simulink model "untitled"  (R2023a)
settings: Solver=daessc  StartTime=0.0  StopTime=15  MaxStep=1e-7  RelTol=1e-3
settings Model: Creator=alexey  LastModifiedBy=alexey

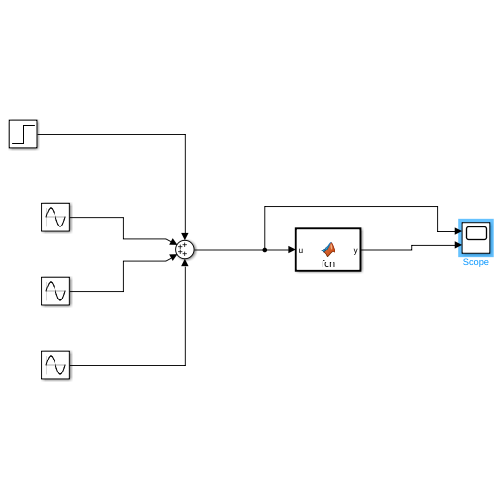
[thumbnail: Simulink's stored preview of the top-level diagram]
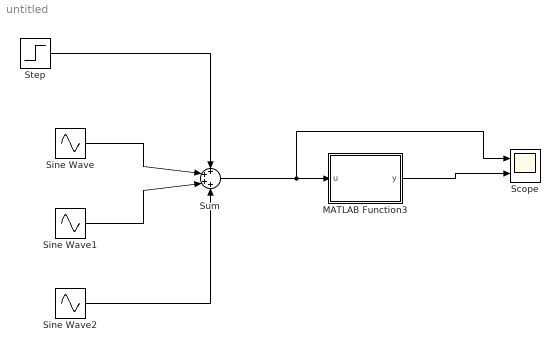
== system untitled ==
  MATLAB Function3 : MATLAB Function  TreatAsAtomicUnit=on  SystemSampleTime=1e-6
  Scope : Scope  NumInputPorts=2
  Sine Wave : Sin  Amplitude=2  Frequency=100*pi  SampleTime=0
  Sine Wave1 : Sin  Amplitude=0.667  Frequency=300*pi  SampleTime=0
  Sine Wave2 : Sin  Amplitude=0.4  Frequency=500*pi  SampleTime=0
  Step : Step  Time=3  SampleTime=0
  Sum : Sum  Inputs=++++
  wires:
  Step/1 -> Sum/1
  Sine Wave/1 -> Sum/2
  Sine Wave1/1 -> Sum/3
  Sine Wave2/1 -> Sum/4
  Sum/1 -> Scope/1, MATLAB Function3/1(u)
  MATLAB Function3/1(y) -> Scope/2

== matlab function untitled/MATLAB Function3 ==
  data: u input; y output
function y = fcn(u)
tetta = 5e-7;

persistent sum;
if(isempty(sum))
    sum = 0;
end


y = tetta * u + (1-tetta)*sum;
sum=y;
